simulink model "sim06b"  (R2020a)
settings: Solver=VariableStepAuto  StartTime=0.0  StopTime=10.0  RelTol=1e-3
values from neighbouring files (symbols this model uses):
  A1 = 10 * 10    (= 100)    [lab06.m]
  a1 = Aw1*sqrt(2*g*(h1max-h2max))/(h1max-h2max)    [lab06.m]
  A2 = A1    (= 100)    [lab06.m]
  a2 = Aw2*sqrt(2*g*h2max)/h2max    [lab06.m]
  czas_skoku = 15    [lab06.m]
  du1 = 0    [lab06.m]
  du2 = 0.1*fwe1max    (= 0.5)    [lab06.m]
  fwe1 = Tab_fwe1(i)    [lab06.m]
  fwe2 = 0.1*fwe1max    (= 0.5)    [lab06.m]
  h10 = fwe1/a1 + h20    [lab06.m]
  h20 = (fwe1 + fwe2)/a2    [lab06.m]
settings Model: Creator=jakub  LastModifiedBy=jakub

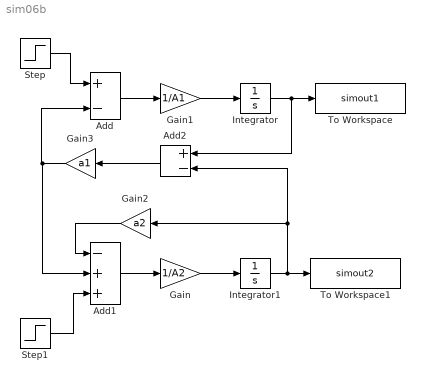
== system sim06b ==
  Add : Sum  Inputs=+-
  Add1 : Sum  Inputs=-++
  Add2 : Sum  Inputs=+-
  Gain : Gain  Gain=1/A2
  Gain1 : Gain  Gain=1/A1
  Gain2 : Gain  Gain=a2
  Gain3 : Gain  Gain=a1
  Integrator : Integrator  InitialCondition=h10
  Integrator1 : Integrator  InitialCondition=h20
  Step : Step  Time=czas_skoku  Before=fwe1  After=fwe1 + du1  SampleTime=0
  Step1 : Step  Time=czas_skoku  Before=fwe2  After=fwe2 + du2  SampleTime=0
  To Workspace : ToWorkspace  VariableName=simout1  SampleTime=-1
  To Workspace1 : ToWorkspace  VariableName=simout2  SampleTime=-1
  wires:
  Gain/1 -> Integrator1/1
  Gain1/1 -> Integrator/1
  Add/1 -> Gain1/1
  Add1/1 -> Gain/1
  Integrator/1 -> Add2/1, To Workspace/1
  Integrator1/1 -> Add2/2, Gain2/1, To Workspace1/1
  Step/1 -> Add/1
  Gain2/1 -> Add1/1
  Step1/1 -> Add1/3
  Gain3/1 -> Add1/2, Add/2
  Add2/1 -> Gain3/1
